simulink model "MobileRobotObstacleAvoidanceWithTarget"  (R2020b)
settings: Solver=VariableStepAuto  StartTime=0.0  StopTime=1000  RelTol=1e-3
values from neighbouring files (symbols this model uses):
  angNoiseSeeds = randi(intmax)    [createEnv.m]    (also in demo.m)
  angNoiseVariance = 0.01^2    (= 0.0001)    [createEnv.m]    (also in demo.m)
  lidarNoiseSeeds = randi(intmax,size(scanAngles))    [createEnv.m]    (also in demo.m)
  lidarNoiseVariance = 0.1^2    (= 0.01)    [createEnv.m]    (also in demo.m)
  mapMatrix = simpleMap    [createEnv.m]    (also in demo.m)
  maxAngSpeed = 0.3    [createEnv.m]    (also in demo.m)
  maxLinSpeed = 0.3    [createEnv.m]    (also in demo.m)
  maxRange = 12    [createEnv.m]    (also in demo.m)
  posNoiseSeeds = randi(intmax,[1, 2])    [createEnv.m]    (also in demo.m)
  posNoiseVariance = 0.1^2    (= 0.01)    [createEnv.m]    (also in demo.m)
  robotTheta = u(3)    [RLAvoidObstaclesTargetResetFcn.m]    (also in createEnv.m = -1.57079632679; demo.m = -1.57079632679)
  robotX = u(1)    [RLAvoidObstaclesTargetResetFcn.m]    (also in createEnv.m = 23; demo.m = 23)
  robotY = u(2)    [RLAvoidObstaclesTargetResetFcn.m]    (also in createEnv.m = 23; demo.m = 23)
  sampleTime = 0.1    [createEnv.m]    (also in demo.m)
  targetTheta = -pi/2    (= -1.57079632679)    [RLAvoidObstaclesTargetResetFcn.m]    (also in createEnv.m; demo.m)
  targetX = 7    [RLAvoidObstaclesTargetResetFcn.m]    (also in createEnv.m; demo.m)
  targetY = 4.5    [RLAvoidObstaclesTargetResetFcn.m]    (also in createEnv.m; demo.m)
libraries: simulink x4, rllib x1, robotmobilelib x1
settings Model: Creator=fan  LastModifiedBy=fanyang

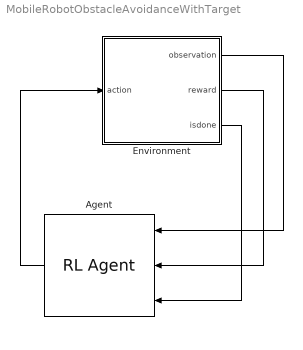
== system MobileRobotObstacleAvoidanceWithTarget ==
  Agent : rllib/RL Agent  Agent=obstacleAvoidanceAgentTarget  ProvideReward=on  ProvideIsDone=on  ProvideCumRwd=off  TreatAsDirectFeedthrough=on  CollectLoggedSignals=on  CollectModelStates=on
  Environment : Subsystem
  wires:
  Agent/1 -> Environment/1(action)
  Environment/3(isdone) -> Agent/3
  Environment/2(reward) -> Agent/2
  Environment/1(observation) -> Agent/1

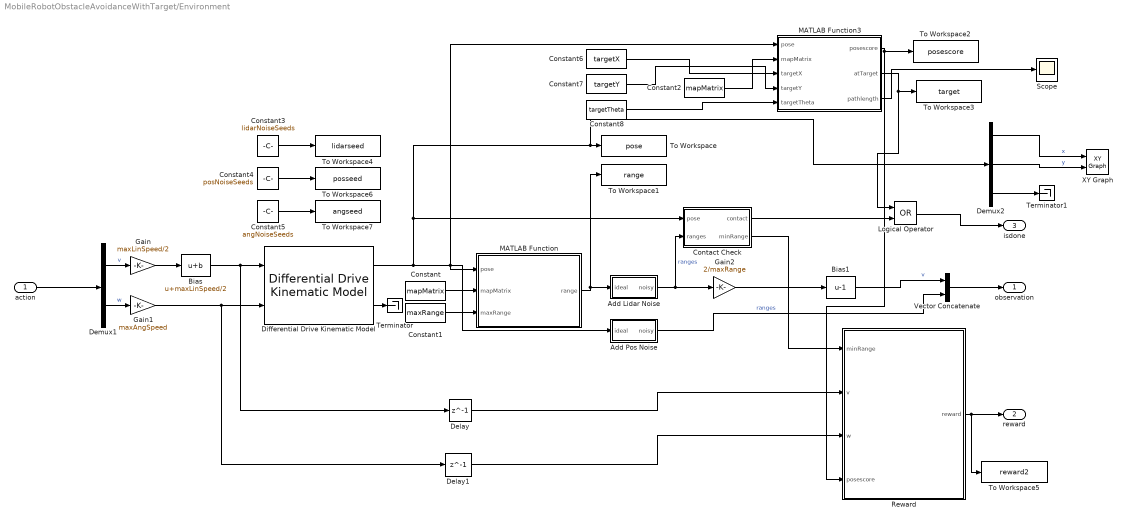
== system MobileRobotObstacleAvoidanceWithTarget/Environment ==
  action : Inport
  Add Lidar Noise : Subsystem
  Add Pos Noise : Subsystem
  Bias : Bias  Bias=maxLinSpeed/2
  Bias1 : Bias  Bias=-1
  Constant : Constant  Value=mapMatrix
  Constant1 : Constant  Value=maxRange
  Constant2 : Constant  Value=mapMatrix
  Constant3 : Constant  Value=lidarNoiseSeeds
  Constant4 : Constant  Value=posNoiseSeeds
  Constant5 : Constant  Value=angNoiseSeeds
  Constant6 : Constant  Value=targetX
  Constant7 : Constant  Value=targetY
  Constant8 : Constant  Value=targetTheta
  Contact Check : Subsystem
  Delay : Delay  DelayLength=1  InitialCondition=0  UseCircularBuffer=on
  Delay1 : Delay  DelayLength=1  InitialCondition=0  UseCircularBuffer=on
  Demux1 : Demux  Outputs=2
  Demux2 : Demux  Outputs=3
  Differential Drive Kinematic Model : robotmobilelib/Differential Drive Kinematic Model  VehicleInputs=Vehicle Speed & Heading Angular Velocity  WheelRadius=0.05  WheelSpeedRange=[-inf inf]  TrackWidth=0.2  InitialState=[robotX; robotY; robotTheta]  SimulateUsing=Code generation
      settings: SourceProductBaseCode=RO
  Gain : Gain  Gain=maxLinSpeed/2
  Gain1 : Gain  Gain=maxAngSpeed
  Gain2 : Gain  Gain=2/maxRange
  Logical Operator : Logic  Operator=OR  AllPortsSameDT=off  OutDataTypeStr=boolean
  MATLAB Function : MATLAB Function  TreatAsAtomicUnit=on
  MATLAB Function3 : MATLAB Function  TreatAsAtomicUnit=on
  Reward : Subsystem
  Scope : Scope
  Terminator : Terminator
  Terminator1 : Terminator
  To Workspace : ToWorkspace  VariableName=pose  SampleTime=-1
      settings: Save2DSignal=2-D array (concatenate along first dimension)
  To Workspace1 : ToWorkspace  VariableName=range  SampleTime=-1
  To Workspace2 : ToWorkspace  VariableName=posescore  SampleTime=-1
      settings: Save2DSignal=2-D array (concatenate along first dimension)
  To Workspace3 : ToWorkspace  VariableName=target  SampleTime=-1
      settings: Save2DSignal=2-D array (concatenate along first dimension)
  To Workspace4 : ToWorkspace  VariableName=lidarseed  SampleTime=-1
      settings: Save2DSignal=2-D array (concatenate along first dimension)
  To Workspace5 : ToWorkspace  VariableName=reward2  SampleTime=-1
      settings: Save2DSignal=2-D array (concatenate along first dimension)
  To Workspace6 : ToWorkspace  VariableName=posseed  SampleTime=-1
      settings: Save2DSignal=2-D array (concatenate along first dimension)
  To Workspace7 : ToWorkspace  VariableName=angseed  SampleTime=-1
      settings: Save2DSignal=2-D array (concatenate along first dimension)
  Vector Concatenate : Concatenate
  XY Graph : simulink/Sinks/XY Graph  xmin=0  xmax=27  ymin=0  ymax=26  st=1
  observation : Outport
  reward : Outport  Port=2
  isdone : Outport  Port=3
  wires:
  Differential Drive Kinematic Model/2 -> Terminator/1
  Constant/1 -> MATLAB Function/2(mapMatrix)
  Differential Drive Kinematic Model/1 -> MATLAB Function/1(pose), MATLAB Function3/1(pose), Add Pos Noise/1(ideal), Demux2/1, To Workspace/1, Contact Check/1(pose)
  action/1 -> Demux1/1
  Bias/1 -> Delay/1, Differential Drive Kinematic Model/1
  Gain1/1 -> Delay1/1, Differential Drive Kinematic Model/2
  MATLAB Function/1(range) -> To Workspace1/1, Add Lidar Noise/1(ideal)
  Contact Check/2(minRange) -> Reward/1(minRange)
  Reward/1(reward) -> To Workspace5/1, reward/1
  Gain2/1 -> Bias1/1
  Constant1/1 -> MATLAB Function/3(maxRange)
  Delay/1 -> Reward/2(v)
  Delay1/1 -> Reward/3(w)
  Demux1/2 -> Gain1/1  "w"
  Gain/1 -> Bias/1
  Demux1/1 -> Gain/1  "v"
  Add Lidar Noise/1(noisy) -> Gain2/1, Contact Check/2(ranges)  "ranges"
  Bias1/1 -> Vector Concatenate/1  "v"
  Add Pos Noise/1(noisy) -> Vector Concatenate/2  "ranges"
  Vector Concatenate/1 -> observation/1
  Constant2/1 -> MATLAB Function3/2(mapMatrix)
  MATLAB Function3/1(posescore) -> Reward/4(posescore), To Workspace2/1
  MATLAB Function3/2(atTarget) -> Logical Operator/1, To Workspace3/1
  Contact Check/1(contact) -> Logical Operator/2
  Logical Operator/1 -> isdone/1
  Demux2/1 -> XY Graph/1  "x"
  Demux2/2 -> XY Graph/2  "y"
  Demux2/3 -> Terminator1/1
  Constant3/1 -> To Workspace4/1
  Constant4/1 -> To Workspace6/1
  Constant5/1 -> To Workspace7/1
  MATLAB Function3/3(pathlength) -> Scope/1
  Constant6/1 -> MATLAB Function3/3(targetX)
  Constant7/1 -> MATLAB Function3/4(targetY)
  Constant8/1 -> MATLAB Function3/5(targetTheta)

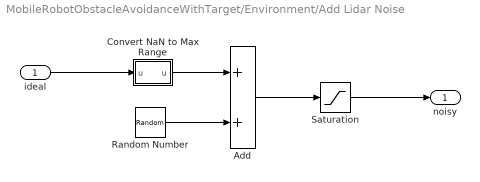
== system MobileRobotObstacleAvoidanceWithTarget/Environment/Add Lidar Noise ==
  ideal : Inport
  Add : Sum
  Convert NaN to Max Range : MATLAB Function  TreatAsAtomicUnit=on
  Random Number : RandomNumber  Variance=lidarNoiseVariance  Seed=lidarNoiseSeeds  SampleTime=sampleTime
  Saturation : Saturate  UpperLimit=inf  LowerLimit=0
  noisy : Outport
  wires:
  Random Number/1 -> Add/2
  Add/1 -> Saturation/1
  Saturation/1 -> noisy/1
  ideal/1 -> Convert NaN to Max Range/1("u ")
  Convert NaN to Max Range/1(u) -> Add/1

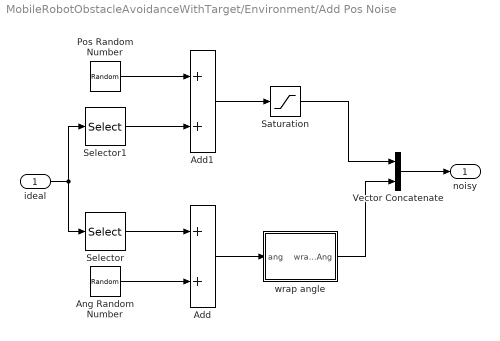
== system MobileRobotObstacleAvoidanceWithTarget/Environment/Add Pos Noise ==
  ideal : Inport
  Add : Sum
  Add1 : Sum
  Ang Random Number : RandomNumber  Variance=angNoiseVariance  Seed=angNoiseSeeds  SampleTime=sampleTime
  Pos Random Number : RandomNumber  Variance=posNoiseVariance  Seed=posNoiseSeeds  SampleTime=sampleTime
  Saturation : Saturate  UpperLimit=inf  LowerLimit=0
  Selector : Selector  InputPortWidth=3  IndexOptions=Index vector (dialog)  Indices=3  OutputSizes=1
  Selector1 : Selector  InputPortWidth=3  IndexOptions=Starting index (dialog)  Indices=1  OutputSizes=2
  Vector Concatenate : Concatenate
  wrap angle : MATLAB Function  TreatAsAtomicUnit=on
  noisy : Outport
  wires:
  ideal/1 -> Selector/1, Selector1/1
  Selector/1 -> Add/1
  Ang Random Number/1 -> Add/2
  Add/1 -> wrap angle/1(ang)
  Selector1/1 -> Add1/2
  Pos Random Number/1 -> Add1/1
  Add1/1 -> Saturation/1
  Saturation/1 -> Vector Concatenate/1
  wrap angle/1(wrapedAng) -> Vector Concatenate/2
  Vector Concatenate/1 -> noisy/1

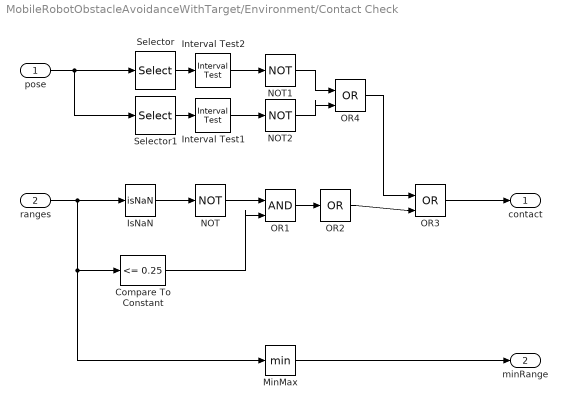
== system MobileRobotObstacleAvoidanceWithTarget/Environment/Contact Check ==
  pose : Inport
  ranges : Inport  Port=2
  Compare To Constant : simulink/Logic and Bit Operations/Compare To Constant  relop=<=  const=0.25  OutDataTypeStr=boolean
  Interval Test1 : simulink/Logic and Bit Operations/Interval Test  IntervalClosedRight=on  uplimit=size(mapMatrix, 1)  IntervalClosedLeft=on  lowlimit=0  OutDataTypeStr=boolean
  Interval Test2 : simulink/Logic and Bit Operations/Interval Test  IntervalClosedRight=on  uplimit=size(mapMatrix, 2)  IntervalClosedLeft=on  lowlimit=0  OutDataTypeStr=boolean
  IsNaN : RelationalOperator  Operator=isNaN  OutDataTypeStr=boolean  RndMeth=Simplest
  MinMax : MinMax
  NOT : Logic  Operator=NOT  IconShape=distinctive  AllPortsSameDT=off  OutDataTypeStr=boolean
  NOT1 : Logic  Operator=NOT  IconShape=distinctive  AllPortsSameDT=off  OutDataTypeStr=boolean
  NOT2 : Logic  Operator=NOT  IconShape=distinctive  AllPortsSameDT=off  OutDataTypeStr=boolean
  OR1 : Logic  IconShape=distinctive  AllPortsSameDT=off  OutDataTypeStr=boolean
  OR2 : Logic  Operator=OR  Inputs=1  IconShape=distinctive  AllPortsSameDT=off  OutDataTypeStr=boolean
  OR3 : Logic  Operator=OR  IconShape=distinctive  AllPortsSameDT=off  OutDataTypeStr=boolean
  OR4 : Logic  Operator=OR  IconShape=distinctive  AllPortsSameDT=off  OutDataTypeStr=boolean
  Selector : Selector  InputPortWidth=3  IndexOptions=Index vector (dialog)  Indices=1  OutputSizes=1
  Selector1 : Selector  InputPortWidth=3  IndexOptions=Index vector (dialog)  Indices=2  OutputSizes=1
  contact : Outport  VectorParamsAs1DForOutWhenUnconnected=off
  minRange : Outport  Port=2  VectorParamsAs1DForOutWhenUnconnected=off
  wires:
  OR1/1 -> OR2/1
  Compare To Constant/1 -> OR1/2
  NOT/1 -> OR1/1
  ranges/1 -> MinMax/1, Compare To Constant/1, IsNaN/1
  IsNaN/1 -> NOT/1
  MinMax/1 -> minRange/1
  OR3/1 -> contact/1
  pose/1 -> Selector/1, Selector1/1
  Selector/1 -> Interval Test2/1
  Selector1/1 -> Interval Test1/1
  OR2/1 -> OR3/2
  NOT1/1 -> OR4/1
  Interval Test1/1 -> NOT2/1
  OR4/1 -> OR3/1
  Interval Test2/1 -> NOT1/1
  NOT2/1 -> OR4/2

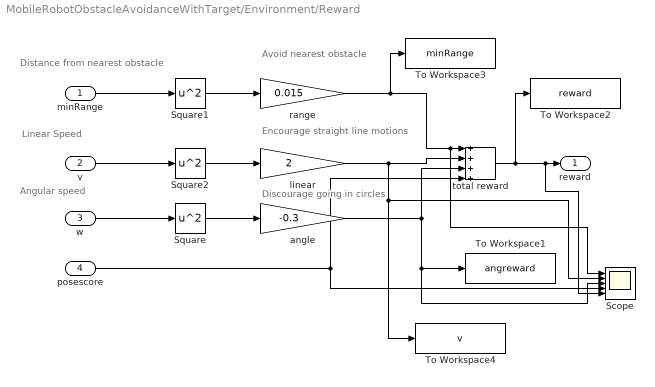
== system MobileRobotObstacleAvoidanceWithTarget/Environment/Reward ==
  note: Discourage going in circles
  note: Encourage straight line motions
  note: Angular speed
  note: Linear Speed
  note: Distance from nearest obstacle
  note: Avoid nearest obstacle
  minRange : Inport
  v : Inport  Port=2
  w : Inport  Port=3
  posescore : Inport  Port=4
  Scope : Scope  NumInputPorts=5
  Square : Math  Operator=square  SignedPower=on  SaturateOnIntegerOverflow=on
  Square1 : Math  Operator=square  SignedPower=on  SaturateOnIntegerOverflow=on
  Square2 : Math  Operator=square  SignedPower=on  SaturateOnIntegerOverflow=on
  To Workspace1 : ToWorkspace  VariableName=angreward  SampleTime=-1
      settings: Save2DSignal=2-D array (concatenate along first dimension)
  To Workspace2 : ToWorkspace  VariableName=reward  SampleTime=-1
      settings: Save2DSignal=2-D array (concatenate along first dimension)
  To Workspace3 : ToWorkspace  VariableName=minRange  SampleTime=-1
      settings: Save2DSignal=2-D array (concatenate along first dimension)
  To Workspace4 : ToWorkspace  VariableName=v  SampleTime=-1
      settings: Save2DSignal=2-D array (concatenate along first dimension)
  angle : Gain  Gain=-0.3
  linear : Gain  Gain=2
  range : Gain  Gain=0.015
  total reward : Sum  Inputs=++++
  reward : Outport  VectorParamsAs1DForOutWhenUnconnected=off
  wires:
  Square/1 -> angle/1
  w/1 -> Square/1
  angle/1 -> To Workspace1/1, Scope/3, total reward/3
  minRange/1 -> Square1/1
  range/1 -> To Workspace3/1, Scope/1, total reward/1
  Square1/1 -> range/1
  v/1 -> Square2/1
  Square2/1 -> linear/1
  linear/1 -> To Workspace4/1, Scope/2, total reward/2
  total reward/1 -> To Workspace2/1, Scope/5, reward/1
  posescore/1 -> total reward/4, Scope/4

== matlab function MobileRobotObstacleAvoidanceWithTarget/Environment/MATLAB Function ==
  settings: updateMethod=DISCRETE
  data: range output size=[7, 1]; pose input size=[3, 1]; mapMatrix input size=[size(mapMatrix, 1), size(mapMatrix, 2)]; maxRange input; mapScale parameter
function range  = RangeSensor(pose, mapMatrix, maxRange, mapScale)
persistent r
if isempty(r)
 r = rangeSensor('HorizontalAngle', [-3*pi/8, 3*pi/8], 'HorizontalAngleResolution', pi/8, 'Range', [0 maxRange]);
end
range = r(pose', binaryOccupancyMap(mapMatrix, mapScale));

%%
% persistent prm
% if isempty(prm)
%     robotRadius = 0.6;
%     mapInflated = copy(binaryOccupancyMap(mapMatrix));
%     inflate(mapInflated,robotRadius);
%     prm = mobileRobotPRM(mapInflated);
%     prm.Map = mapInflated;
%     prm.NumNodes = 500;
%     prm.ConnectionDistance = 2;
% end
% 
% path = findpath(prm, pose(1:2)', [22, 3]);
% % path = findpath(prm, [5, 22], [22, 3]);
% 
% path1 = path(1:end-1, :);
% path2 = path(2:end, :);
% diff = (path1 - path2).^2;
% pair_dis = sqrt(sum(diff,2));
% pl = sum(pair_dis);
end

== matlab function MobileRobotObstacleAvoidanceWithTarget/Environment/Add Lidar Noise/Convert NaN to Max Range ==
  data: u input; u output; maxRange parameter
function u = removeNans(u,maxRange)

u(isnan(u)) = maxRange;

== matlab function MobileRobotObstacleAvoidanceWithTarget/Environment/Add Pos Noise/wrap angle ==
  data: ang input; wrapedAng output
function wrapedAng = fcn(ang)
% wrapedAng = wrapTo2Pi(ang);

abs_ang = abs(ang);

if abs_ang > 2*pi
    Ang = mod(abs_ang./pi,2) .* pi;
else
    Ang = abs_ang;
end

if ang < 0
    wrapedAng = 2*pi - Ang;
else
    wrapedAng = Ang;
end

end

== matlab function MobileRobotObstacleAvoidanceWithTarget/Environment/MATLAB Function3 ==
  settings: updateMethod=DISCRETE
  data: pose input size=[3, 1]; mapMatrix input size=[size(mapMatrix, 1), size(mapMatrix, 2)]; posescore output; atTarget output; pathlength output; targetX input; targetY input; targetTheta input
function [posescore, atTarget,pathlength] = poseEval(pose, mapMatrix, targetX, targetY, targetTheta)

persistent prm
if isempty(prm)
    map = binaryOccupancyMap(mapMatrix);
    prm = mobileRobotPRM(map);
    prm.NumNodes = 1000;
    prm.ConnectionDistance = 3;
end

%% compute distance to target
path = findpath(prm, [pose(1), pose(2)], [targetX, targetY]);

path1 = path(1:end-1, :);
path2 = path(2:end, :);
diff = (path1 - path2).^2;
pair_dis = sqrt(sum(diff,2));
pathlength = sum(pair_dis);
cos_dist = cos(pose(3)-targetTheta);
%% compute path score    

posescore = 6 / pathlength;

if pathlength < 2
    posescore = 3*posescore + 5 * cos_dist;
end
%% In case that no path is found
if pathlength == 0
    posescore = 0.1;
end


%% stopping criteria 
atTarget = false;
% if pathlength <= 0.5 && 1- cos_dist <= 0.038
%     atTarget = true;
%     pathscore = 1000;
% end

if pathlength <= 1
    atTarget = true;
    posescore = 1000;
end


end
